simulink model "IP_DLQ"  (R2022b)
settings: Solver=ode15s  StartTime=0.0  StopTime=t_sim  RelTol=1e-3
undefined symbols (not defined in the file): b1, b2, deltaT, etag, etam, g, Kgi, Klift, km, kt, Lb, liftFun, Lp, mb, mp, Rm, xbar
settings Model: Creator=vince  LastModifiedBy=vince

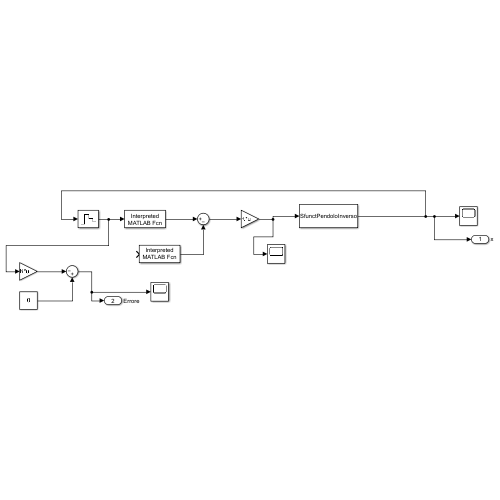
[thumbnail: Simulink's stored preview of the top-level diagram]
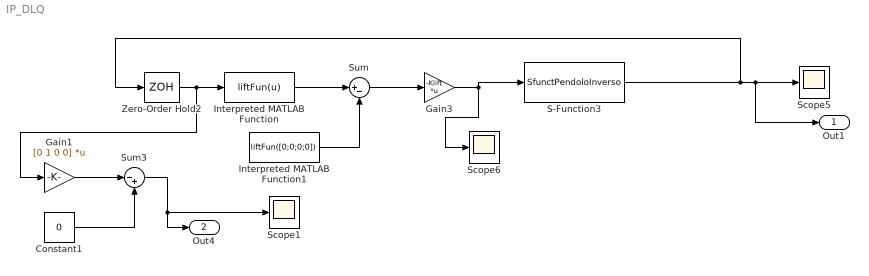
== system IP_DLQ ==
  Constant1 : Constant  Value=0
  Gain1 : Gain  Gain=[0 1 0 0]  Multiplication=Matrix(K*u)
  Gain3 : Gain  Gain=-Klift  Multiplication=Matrix(K*u)
  Interpreted MATLAB Function : MATLABFcn  MATLABFcn=liftFun(u)
  Interpreted MATLAB Function1 : MATLABFcn  MATLABFcn=liftFun([0;0;0;0])
  S-Function3 : S-Function  FunctionName=SfunctPendoloInverso  Parameters=xbar,mb,mp,Lb,Lp,b1,b2,g,Rm,kt,km,Kgi,etag,etam  SFunctionDeploymentMode=off  EnableBusSupport=off
  Scope1 : Scope
  Scope5 : Scope
  Scope6 : Scope
  Sum : Sum  Inputs=|+-
  Sum3 : Sum  Inputs=|-+
  Zero-Order Hold2 : ZeroOrderHold  SampleTime=deltaT
  Out1 : Outport  SignalName=x
  Out4 : Outport  Port=2  SignalName=Errore
  wires:
  Constant1/1 -> Sum3/2
  Sum/1 -> Gain3/1
  Gain1/1 -> Sum3/1
  Gain3/1 -> S-Function3/1, Scope6/1
  Interpreted MATLAB Function/1 -> Sum/1
  Zero-Order Hold2/1 -> Gain1/1, Interpreted MATLAB Function/1
  Interpreted MATLAB Function1/1 -> Sum/2
  Sum3/1 -> Scope1/1, Out4/1
  S-Function3/1 -> Out1/1, Scope5/1, Zero-Order Hold2/1
